simulink model "history_stack"  (Simulink 7.3)
settings: Solver=FixedStepDiscrete  StartTime=0.0  StopTime=10.0  FixedStep=1  RelTol=1e-3
libraries: simulink x2, dspbuff3 x1
settings Model: Creator=alp.marangoz  LastModifiedBy=alp.marangoz

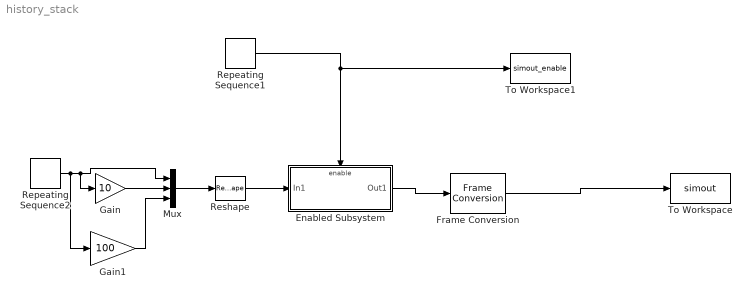
== system history_stack ==
  Enabled Subsystem : Subsystem  TreatAsAtomicUnit=on
  Frame Conversion : FrameConversion  OutFrame=Sample-based
  Gain : Gain  Gain=10  ParameterDataType=fixdt(1, 16)  ParameterScaling=2^0  OutDataType=fixdt(1, 16)  OutScaling=2^0
  Gain1 : Gain  Gain=100  ParameterDataType=fixdt(1, 16)  ParameterScaling=2^0  OutDataType=fixdt(1, 16)  OutScaling=2^0
  Mux : Mux  Inputs=3
  Repeating Sequence1 : simulink/Sources/Repeating Sequence  SystemSampleTime=-1  rep_seq_t=[0 1 2 3 4 5 6 7 8 9 10]  rep_seq_y=[1 1 1 0 0 1 1 1 1 0 0]
  Repeating Sequence2 : simulink/Sources/Repeating Sequence  SystemSampleTime=-1  rep_seq_t=[0 1 2 3 4 5 6 7 8 9 10]  rep_seq_y=0:10
  Reshape : Reshape  OutputDimensionality=Column vector (2-D)
  To Workspace : ToWorkspace  VariableName=simout  SampleTime=-1  SaveFormat=Structure
  To Workspace1 : ToWorkspace  VariableName=simout_enable  SampleTime=-1  SaveFormat=Structure
  wires:
  Mux/1 -> Reshape/1
  Repeating Sequence1/1 -> Enabled Subsystem/Enable, To Workspace1/1
  Enabled Subsystem/1(Out1) -> Frame Conversion/1
  Frame Conversion/1 -> To Workspace/1
  Repeating Sequence2/1 -> Mux/1, Gain/1, Gain1/1
  Gain/1 -> Mux/2
  Gain1/1 -> Mux/3
  Reshape/1 -> Enabled Subsystem/1(In1)

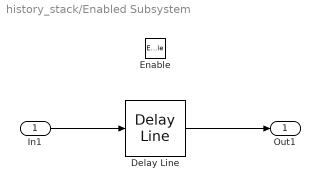
== system history_stack/Enabled Subsystem ==
  In1 : Inport  OutDataType=fixdt(1, 16)  OutScaling=2^0
  Enable : EnablePort
  Delay Line : dspbuff3/Delay Line  siz=10  ic=0  directfeed=on  enable_output=off  hold_output=off
  Out1 : Outport  OutDataType=fixdt(1, 16)  OutScaling=2^0
  wires:
  In1/1 -> Delay Line/1
  Delay Line/1 -> Out1/1
